simulink model "TRAS_process_"  (R2024b)
settings: Solver=FixedStepAuto  StartTime=0.0  StopTime=stop_time  FixedStep=sampling_time  RelTol=1e-3
values from neighbouring files (symbols this model uses):
  A = 0.0552    [momentsOfInertia.m]
  B = 0.0599    [momentsOfInertia.m]
  C = 0.0084    [momentsOfInertia.m]
  D = (mmr + mms + mm / 3) * lm^2 + (mtr + mts + mt / 3) * lt^2    (= 0.0224143186667)    [momentsOfInertia.m]
  F = mms * rms^2 + mts * rts^2    (= 0.002355075)    [momentsOfInertia.m]
  Fh = [-2.6*1e-20, 4.1*1e-17, 3.2*1e-12, -7.3*1e-9, 2.1*1e-5, 0]    [thrustForcesDependencies.m]
  Fv = [-1.8*1e-18, -8.8*1e-16, 4.1*1e-11, 2.7*1e-8, 3.5*1e-5, 0]    [thrustForcesDependencies.m]
  g = 9.81    [TRAS_closed_loop.m]    (also in TRAS_controller.m; TRAS_process.m)
  Jv = D + E + F    (= 0.0253918936667)    [momentsOfInertia.m]
  Kh = [-Kdecline / 4000^2, 0, Kpeak]    [thrustForcesDependencies.m]
  Kv = [-Kdecline / 4000^2, 0, Kpeak]    [thrustForcesDependencies.m]
  lm = 0.202    [momentsOfInertia.m]
  lt = 0.216    [momentsOfInertia.m]
  sampling_time = 1e-2    (= 0.01)    [TRAS_closed_loop.m]    (also in TRAS_controller.m; TRAS_process.m; identification.m)
  Th = [-Tdecline / 4000^2, 0, Tpeak]    [thrustForcesDependencies.m]
  Tv = [-Tdecline / 4000^2, 0, Tpeak]    [thrustForcesDependencies.m]
libraries: simulink x2
settings Model: Creator=Codrin  LastModifiedBy=Codrin

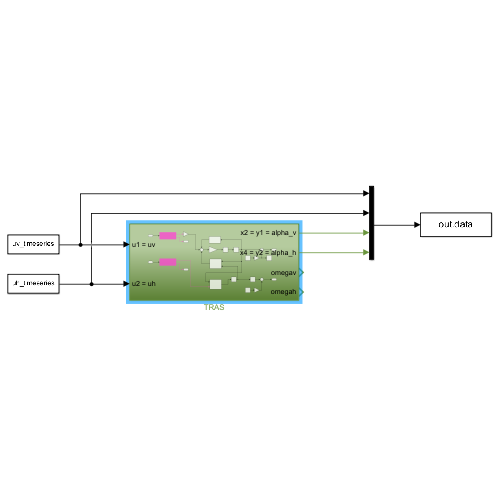
[thumbnail: Simulink's stored preview of the top-level diagram]
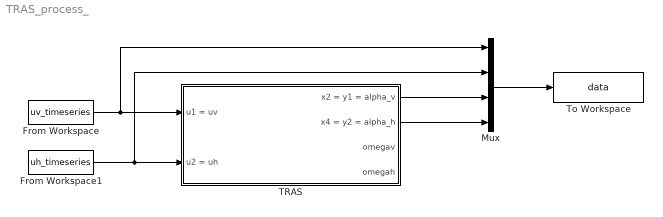
== system TRAS_process_ ==
  From Workspace : FromWorkspace  VariableName=uv_timeseries
  From Workspace1 : FromWorkspace  VariableName=uh_timeseries
  Mux : Mux
  TRAS : Subsystem
  To Workspace : ToWorkspace  VariableName=data  SaveFormat=Timeseries  SampleTime=-1
  wires:
  From Workspace/1 -> TRAS/1(u1 = uv), Mux/1
  From Workspace1/1 -> TRAS/2(u2 = uh), Mux/2
  Mux/1 -> To Workspace/1
  TRAS/1(x2 = y1 = alpha_v) -> Mux/3
  TRAS/2(x4 = y2 = alpha_h) -> Mux/4

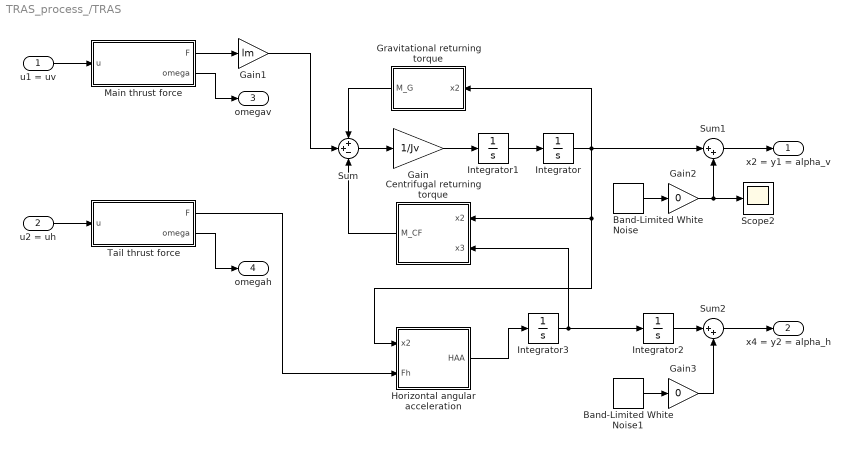
== system TRAS_process_/TRAS ==
  u1 = uv : Inport
  u2 = uh : Inport  Port=2
  Band-Limited White Noise : simulink/Sources/Band-Limited White Noise  Cov=[0.01]  Ts=sampling_time  seed=[23341]
  Band-Limited White Noise1 : simulink/Sources/Band-Limited White Noise  Cov=[0.01]  Ts=sampling_time  seed=[23341]
  Centrifugal returning torque : MATLAB Function  TreatAsAtomicUnit=on
  Gain : Gain  Gain=1/Jv
  Gain1 : Gain  Gain=lm
  Gain2 : Gain  Gain=0
  Gain3 : Gain  Gain=0
  Gravitational returning torque : MATLAB Function  TreatAsAtomicUnit=on
  Horizontal angular acceleration : MATLAB Function  TreatAsAtomicUnit=on
  Integrator{,1..3} (4 alike) : Integrator
  Main thrust force : Subsystem
  Scope2 : Scope
  Sum : Sum  Inputs=++-
  Sum1 : Sum  Inputs=|++
  Sum2 : Sum  Inputs=|++
  Tail thrust force : Subsystem
  x2 = y1 = alpha_v : Outport
  x4 = y2 = alpha_h : Outport  Port=2
  omegav : Outport  Port=3
  omegah : Outport  Port=4
  wires:
  u1 = uv/1 -> Main thrust force/1(u)
  Integrator/1 -> Sum1/1, Horizontal angular acceleration/1(x2), Centrifugal returning torque/1(x2), Gravitational returning torque/1(x2)
  Integrator1/1 -> Integrator/1
  Gain/1 -> Integrator1/1
  Sum/1 -> Gain/1
  Gravitational returning torque/1(M_G) -> Sum/1
  Main thrust force/1(F) -> Gain1/1
  Gain1/1 -> Sum/2
  Centrifugal returning torque/1(M_CF) -> Sum/3
  Integrator3/1 -> Integrator2/1, Centrifugal returning torque/2(x3)
  u2 = uh/1 -> Tail thrust force/1(u)
  Tail thrust force/1(F) -> Horizontal angular acceleration/2(Fh)
  Horizontal angular acceleration/1(HAA) -> Integrator3/1
  Sum1/1 -> x2 = y1 = alpha_v/1
  Sum2/1 -> x4 = y2 = alpha_h/1
  Integrator2/1 -> Sum2/1
  Band-Limited White Noise1/1 -> Gain3/1
  Gain3/1 -> Sum2/2
  Band-Limited White Noise/1 -> Gain2/1
  Gain2/1 -> Scope2/1, Sum1/2
  Main thrust force/2(omega) -> omegav/1
  Tail thrust force/2(omega) -> omegah/1

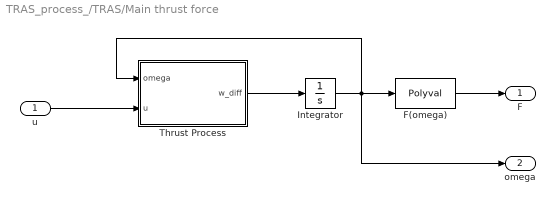
== system TRAS_process_/TRAS/Main thrust force ==
  u : Inport
  F(omega) : Polyval  Coefs=Fv
  Integrator : Integrator
  Thrust Process : MATLAB Function  TreatAsAtomicUnit=on
  F : Outport
  omega : Outport  Port=2
  wires:
  F(omega)/1 -> F/1
  Integrator/1 -> omega/1, Thrust Process/1(omega), F(omega)/1
  Thrust Process/1(w_diff) -> Integrator/1
  u/1 -> Thrust Process/2(u)

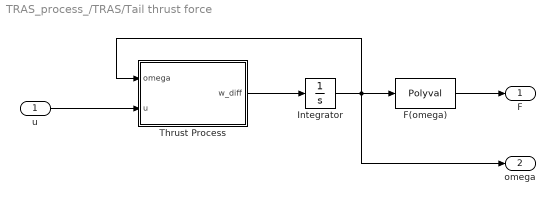
== system TRAS_process_/TRAS/Tail thrust force ==
  u : Inport
  F(omega) : Polyval  Coefs=Fh
  Integrator : Integrator
  Thrust Process : MATLAB Function  TreatAsAtomicUnit=on
  F : Outport
  omega : Outport  Port=2
  wires:
  u/1 -> Thrust Process/2(u)
  Thrust Process/1(w_diff) -> Integrator/1
  Integrator/1 -> F(omega)/1, Thrust Process/1(omega), omega/1
  F(omega)/1 -> F/1

== matlab function TRAS_process_/TRAS/Centrifugal returning torque ==
  data: x2 input; M_CF output; x3 input; L parameter
function M_CF = M_CF(x2, x3, L)

M_CF = x3^2 / 2 * L * sin(2 * x2);

== matlab function TRAS_process_/TRAS/Gravitational returning torque ==
  data: x2 input; M_G output; g parameter; A parameter; B parameter; C parameter
function M_G = M_G(x2, g, A, B, C)

M_G = g * ((A - B) * cos(x2) - C * sin(x2));

== matlab function TRAS_process_/TRAS/Horizontal angular acceleration ==
  data: x2 input; Fh input; HAA output; lt parameter; D parameter; E parameter; F parameter
function HAA = HAA(x2, Fh, lt, D, E, F)

HAA = lt * Fh * cos(x2) / (D * cos(x2)^2 + E * sin(x2)^2 + F);

== matlab function TRAS_process_/TRAS/Main thrust force/Thrust Process ==
  data: omega input; u input; w_diff output; Tv parameter; Kv parameter
function w_diff = thrustProcess(omega, u, Tv, Kv)

w_diff = -1/polyval(Tv, omega)*omega + polyval(Kv, omega) / polyval(Tv, omega)*u;

== matlab function TRAS_process_/TRAS/Tail thrust force/Thrust Process ==
  data: omega input; u input; w_diff output; Th parameter; Kh parameter
function w_diff = thrustProcess(omega, u, Th, Kh)

w_diff = -1/polyval(Th, omega)*omega + polyval(Kh, omega) / polyval(Th, omega)*u;
